simulink model "clc_sldv_m6"  (R2020b)
settings: Solver=ode3  StartTime=0.0  StopTime=simTime  FixedStep=0.01  RelTol=1e-6  AbsTol=1e-7
model workspace (MATLAB code in the model file):
  | % Load initial conditions and other information
  | 
  | load sldemo_clutchparam;
undefined symbols (not defined in the file): be, bv, DiscIntNeverNeededParam, Ie, Iv, muk, mus, R
Description:
  | Building a Clutch Lock-Up Model
  | 
  | This example demonstrates the use of Simulink to model and simulate a
  | rotating clutch system. Although modeling a clutch system is difficult
  | because of topological changes in the system dynamics during lockup, this
  | example shows how Simulinks enabled subsystems feature easily handles
  | such problems. We illustrate how to employ important Simulink modeling
  | concepts in the creation of the clutch simulation. Designers can apply
  | these concepts to many models with strong discontinuities and constraints
  | that may change dynamically.
  | 
  | In the demonstration, we use enabled subsystems to build the clutch
  | model. Two enabled subsystems model the clutch dynamics in either the
  | locked or unlocked position. After running the simulation, a GUI opens.
  | Checking any of the boxes on the GUI produces a plot of any of the
  | selected variables (versus time).
settings Model: ExtModeTrigMode=oneshot  ExtModeArmWhenConnect=off  ExtModeAutoUpdateStatusClock=off  Creator=The MathWorks Inc.  LastModifiedBy=Xiao Ling
settings SolverCC: AutoScaleAbsTol=off
settings DataIOCC: ExternalInput=externalinputdata  InitialState=[]  SaveFormat=Array  SignalLoggingSaveFormat=ModelDataLogs  SignalLogging=off  DSMLogging=off  ReturnWorkspaceOutputs=off  StateSaveName=x  SignalLoggingName=sldemo_clutch_output
settings OptimizationCC: BlockReduction=off  BooleanDataType=off  ExpressionDepthLimit=2147483647  InitFltsAndDblsToZero=on  LifeSpan=inf  BufferReusableBoundary=off
settings DebuggingCC: SaveWithParameterizedLinksMsg=none  UnderspecifiedInitializationDetection=Classic  MergeDetectMultiDrivingBlocksExec=none  SignalResolutionControl=TryResolveAllWithWarning  MultiTaskDSMMsg=warning  MultiTaskCondExecSysMsg=none  SigSpecEnsureSampleTimeMsg=none  IntegerOverflowMsg=none  FcnCallInpInsideContextMsg=warning  BusObjectLabelMismatch=none  StateNameClashWarn=warning  SFUnexpectedBacktrackingDiag=warning  SFNoUnconditionalDefaultTransitionDiag=warning  SFExecutionAtInitializationDiag=none  IntegerSaturationMsg=none  ArithmeticOperatorsInVariantConditions=warning
settings HardwareCC: ProdBitPerPointer=32  ProdBitPerSizeT=32  ProdBitPerPtrDiffT=32  ProdLargestAtomicFloat=None  ProdIntDivRoundTo=Undefined  ProdEndianess=Unspecified  ProdWordSize=32  ProdHWDeviceType=32-bit Generic  TargetUnknown=on
settings ModelReferenceCC: PropagateSignalLabelsOutOfModel=off
settings CodeAppCC: StateflowObjectComments=on
settings GRTTargetCC: TargetFcnLib=ansi_tfl_tmw.mat  TargetLangStandard=C89/C90 (ANSI)  CombineOutputUpdateFcns=off  GRTInterface=on
settings ConfigComp: CovMetricSettings=d  CovSaveCumulativeToWorkspaceVar=on  CovSaveSingleToWorkspaceVar=on  DVMaxProcessTime=600  DVParameters=on  DVModelCoverageObjectives=Decision  DVMaxTestCaseSteps=500  DVTestSuiteOptimization=CombinedObjectives  DVDetectActiveLogic=on  DVDetectOutOfBounds=on  DVSaveHarnessModel=on  DVSaveReport=on

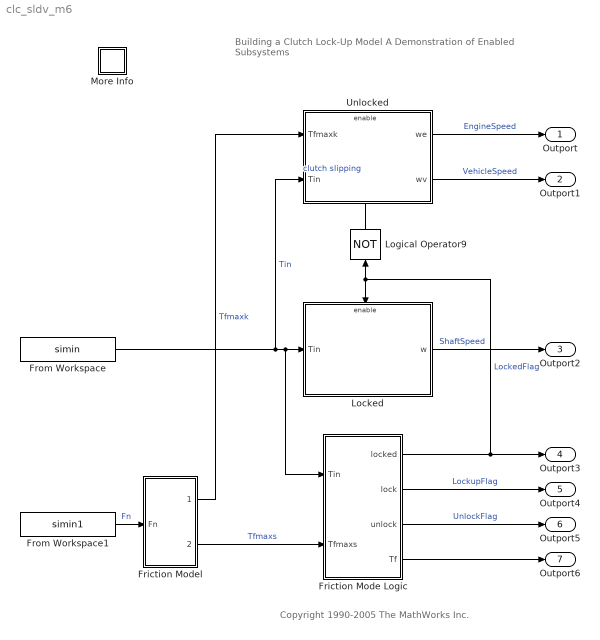
== system clc_sldv_m6 ==
  note: Building a Clutch Lock-Up Model
      | A Demonstration of Enabled Subsystems
  note: Copyright 1990-2005 The MathWorks Inc.
  Friction Model : Subsystem
  Friction Mode Logic : Subsystem
      mask Display: plot([-3 1 1 3 -1 -1],[-1 -1 1 1 1 -1],-4,-5,4,5)
  From Workspace : FromWorkspace  VariableName=simin
  From Workspace1 : FromWorkspace  VariableName=simin1
  Locked : Subsystem  TreatAsAtomicUnit=on
      mask Display: plot(-1,-6,6,12,[0 3],[3 3],[3 1 1 3], [1 1 5 5],[2 4 4 2],[4 4 2 2],[4 5],[3 3])
  Logical Operator9 : Logic  Operator=NOT  Inputs=1  IconShape=distinctive
  More Info : Subsystem
      settings: OpenFcn=showdemo(bdroot(gcb))
      mask Display: disp('?')
  Unlocked : Subsystem  TreatAsAtomicUnit=on
      mask Display: plot(-1,-2,6,8,[0 3],[3 3],[3 1 1 3], [1 1 5 5],[2 4 4 2],[4 4 2 2],[4 5],[3 3])
  Outport : Outport
  Outport1 : Outport  Port=2
  Outport2 : Outport  Port=3
  Outport3 : Outport  Port=4
  Outport4 : Outport  Port=5
  Outport5 : Outport  Port=6
  Outport6 : Outport  Port=7
  wires:
  Friction Mode Logic/3(unlock) -> Outport5/1  "UnlockFlag"
  From Workspace/1 -> Locked/1(Tin), Friction Mode Logic/1(Tin), Unlocked/2(Tin)  "Tin"
  Friction Model/1(Tfmaxk) -> Unlocked/1(Tfmaxk)  "Tfmaxk"
  Unlocked/2(wv) -> Outport1/1  "VehicleSpeed"
  Unlocked/1(we) -> Outport/1  "EngineSpeed"
  Friction Mode Logic/1(locked) -> Outport3/1, Logical Operator9/1, Locked/Enable  "LockedFlag"
  Friction Mode Logic/2(lock) -> Outport4/1  "LockupFlag"
  Friction Mode Logic/4(Tf) -> Outport6/1
  Locked/1(w) -> Outport2/1  "ShaftSpeed"
  Logical Operator9/1 -> Unlocked/Enable  "clutch slipping"
  Friction Model/2(Tfmaxs) -> Friction Mode Logic/2(Tfmaxs)  "Tfmaxs"
  From Workspace1/1 -> Friction Model/1(Fn)  "Fn"

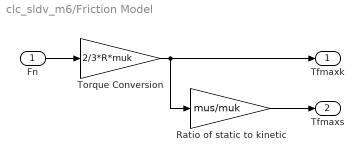
== system clc_sldv_m6/Friction Model ==
  Fn : Inport
  Ratio of static to kinetic : Gain  Gain=mus/muk  SaturateOnIntegerOverflow=on  OutDataTypeStr=Inherit: Same as input  ParamDataTypeStr=Inherit: Same as input
  Torque Conversion : Gain  Gain=2/3*R*muk  SaturateOnIntegerOverflow=on  OutDataTypeStr=Inherit: Same as input  ParamDataTypeStr=Inherit: Same as input
  Tfmaxk : Outport  InitialOutput=0
  Tfmaxs : Outport  Port=2  InitialOutput=0
  wires:
  Torque Conversion/1 -> Tfmaxk/1, Ratio of static to kinetic/1
  Fn/1 -> Torque Conversion/1
  Ratio of static to kinetic/1 -> Tfmaxs/1

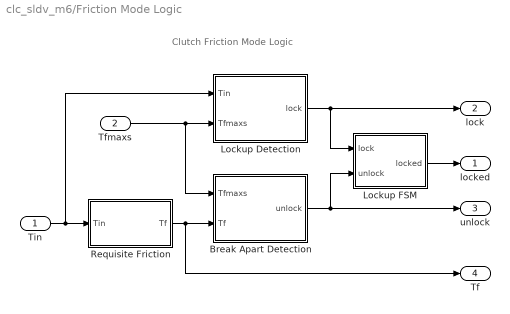
== system clc_sldv_m6/Friction Mode Logic ==
  note: Clutch Friction Mode Logic
  Tin : Inport
  Tfmaxs : Inport  Port=2
  Break Apart Detection : Subsystem
  Lockup Detection : Subsystem
  Lockup FSM : Subsystem
  Requisite Friction : Subsystem
  locked : Outport  InitialOutput=0
  lock : Outport  Port=2  InitialOutput=0
  unlock : Outport  Port=3  InitialOutput=0
  Tf : Outport  Port=4  InitialOutput=0
  wires:
  Tin/1 -> Lockup Detection/1(Tin), Requisite Friction/1(Tin)
  Tfmaxs/1 -> Lockup Detection/2(Tfmaxs), Break Apart Detection/1(Tfmaxs)
  Requisite Friction/1(Tf) -> Break Apart Detection/2(Tf), Tf/1
  Break Apart Detection/1(unlock) -> Lockup FSM/2(unlock), unlock/1
  Lockup Detection/1(lock) -> Lockup FSM/1(lock), lock/1
  Lockup FSM/1(locked) -> locked/1

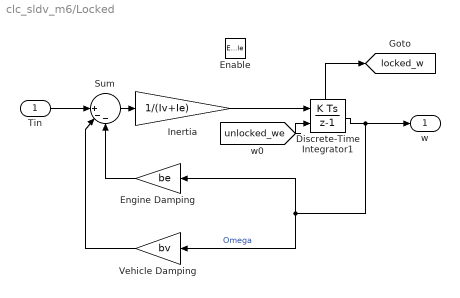
== system clc_sldv_m6/Locked ==
  Tin : Inport
  Enable : EnablePort  StatesWhenEnabling=reset
  Discrete-Time Integrator1 : DiscreteIntegrator  InitialConditionSource=external  ShowStatePort=on  ICPrevOutput=DiscIntNeverNeededParam  ICPrevScaledInput=DiscIntNeverNeededParam
  Engine Damping : Gain  Gain=be  SaturateOnIntegerOverflow=on  OutDataTypeStr=Inherit: Same as input  ParamDataTypeStr=Inherit: Same as input
  Inertia : Gain  Gain=1/(Iv+Ie)  SaturateOnIntegerOverflow=on  OutDataTypeStr=Inherit: Same as input  ParamDataTypeStr=Inherit: Same as input
  Sum : Sum  Inputs=||+--  InputSameDT=on  SaturateOnIntegerOverflow=on  OutDataTypeStr=Inherit: Same as first input
  Vehicle Damping : Gain  Gain=bv  SaturateOnIntegerOverflow=on  OutDataTypeStr=Inherit: Same as input  ParamDataTypeStr=Inherit: Same as input
  w : Outport  InitialOutput=0
  tag scope: locked_w=global
  wires:
  [unlocked_we] -> Discrete-Time Integrator1/2
  Discrete-Time Integrator1/State -> [locked_w]
  Sum/1 -> Inertia/1
  Tin/1 -> Sum/1
  Discrete-Time Integrator1/1 -> w/1, Engine Damping/1, Vehicle Damping/1  "Omega"
  Engine Damping/1 -> Sum/3
  Inertia/1 -> Discrete-Time Integrator1/1
  Vehicle Damping/1 -> Sum/2

== system clc_sldv_m6/More Info ==

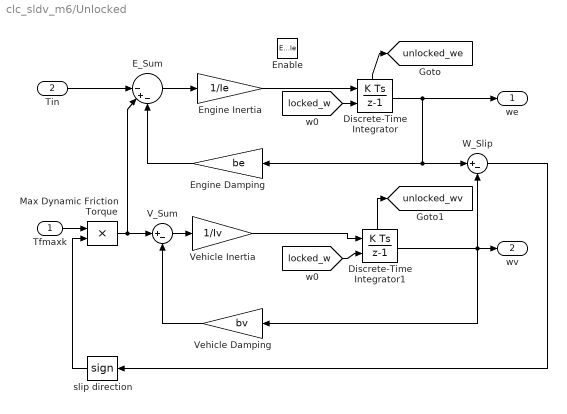
== system clc_sldv_m6/Unlocked ==
  Tfmaxk : Inport
  Tin : Inport  Port=2
  Enable : EnablePort  StatesWhenEnabling=reset
  Discrete-Time Integrator : DiscreteIntegrator  InitialConditionSource=external  ShowStatePort=on  ICPrevOutput=DiscIntNeverNeededParam  ICPrevScaledInput=DiscIntNeverNeededParam
  Discrete-Time Integrator1 : DiscreteIntegrator  InitialConditionSource=external  ShowStatePort=on  ICPrevOutput=DiscIntNeverNeededParam  ICPrevScaledInput=DiscIntNeverNeededParam
  E_Sum : Sum  Inputs=||-+-  InputSameDT=on  SaturateOnIntegerOverflow=on  OutDataTypeStr=Inherit: Same as first input
  Engine Damping : Gain  Gain=be  SaturateOnIntegerOverflow=on  OutDataTypeStr=Inherit: Same as input  ParamDataTypeStr=Inherit: Same as input
  Engine Inertia : Gain  Gain=1/Ie  SaturateOnIntegerOverflow=on  OutDataTypeStr=Inherit: Same as input  ParamDataTypeStr=Inherit: Same as input
  Max Dynamic Friction Torque : Product  InputSameDT=on  RndMeth=Zero  SaturateOnIntegerOverflow=on  OutDataTypeStr=Inherit: Same as first input
  V_Sum : Sum  Inputs=|+-  InputSameDT=on  SaturateOnIntegerOverflow=on  OutDataTypeStr=Inherit: Same as first input
  Vehicle Damping : Gain  Gain=bv  SaturateOnIntegerOverflow=on  OutDataTypeStr=Inherit: Same as input  ParamDataTypeStr=Inherit: Same as input
  Vehicle Inertia : Gain  Gain=1/Iv  SaturateOnIntegerOverflow=on  OutDataTypeStr=Inherit: Same as input  ParamDataTypeStr=Inherit: Same as input
  W_Slip : Sum  Inputs=|+-  InputSameDT=on  SaturateOnIntegerOverflow=on  OutDataTypeStr=Inherit: Same as first input
  slip direction : Signum
  we : Outport  InitialOutput=0
  wv : Outport  Port=2  InitialOutput=0
  tag scope: unlocked_we=global, unlocked_wv=global
  wires:
  V_Sum/1 -> Vehicle Inertia/1
  Vehicle Damping/1 -> V_Sum/2
  Max Dynamic Friction Torque/1 -> V_Sum/1, E_Sum/2
  Tfmaxk/1 -> Max Dynamic Friction Torque/1
  slip direction/1 -> Max Dynamic Friction Torque/2
  W_Slip/1 -> slip direction/1
  Discrete-Time Integrator/State -> [unlocked_we]
  Engine Inertia/1 -> Discrete-Time Integrator/1
  E_Sum/1 -> Engine Inertia/1
  Engine Damping/1 -> E_Sum/3
  Discrete-Time Integrator/1 -> we/1, Engine Damping/1, W_Slip/1
  [locked_w] -> Discrete-Time Integrator/2
  Tin/1 -> E_Sum/1
  Discrete-Time Integrator1/State -> [unlocked_wv]
  [locked_w] -> Discrete-Time Integrator1/2
  Vehicle Inertia/1 -> Discrete-Time Integrator1/1
  Discrete-Time Integrator1/1 -> wv/1, W_Slip/2, Vehicle Damping/1

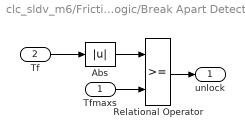
== system clc_sldv_m6/Friction Mode Logic/Break Apart Detection ==
  Tfmaxs : Inport
  Tf : Inport  Port=2
  Abs : Abs  SaturateOnIntegerOverflow=on
  Relational Operator : RelationalOperator  RndMeth=Nearest  InputSameDT=on
  unlock : Outport  InitialOutput=0
  wires:
  Tf/1 -> Abs/1
  Relational Operator/1 -> unlock/1
  Abs/1 -> Relational Operator/1
  Tfmaxs/1 -> Relational Operator/2

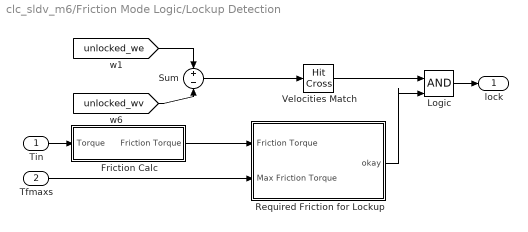
== system clc_sldv_m6/Friction Mode Logic/Lockup Detection ==
  Tin : Inport
  Tfmaxs : Inport  Port=2
  Friction Calc : Subsystem
  Logic : Logic  IconShape=distinctive
  Required Friction for Lockup : Subsystem
  Sum : Sum  Inputs=+-  InputSameDT=on  SaturateOnIntegerOverflow=on  OutDataTypeStr=Inherit: Same as first input
  Velocities Match : HitCross
  lock : Outport  InitialOutput=0
  wires:
  Friction Calc/1(Friction Torque) -> Required Friction for Lockup/1(Friction Torque)
  Tfmaxs/1 -> Required Friction for Lockup/2(Max Friction Torque)
  Velocities Match/1 -> Logic/1
  Logic/1 -> lock/1
  Required Friction for Lockup/1(okay) -> Logic/2
  [unlocked_we] -> Sum/1
  [unlocked_wv] -> Sum/2
  Sum/1 -> Velocities Match/1
  Tin/1 -> Friction Calc/1(Torque)

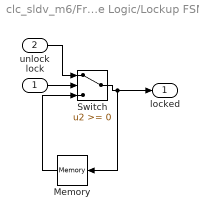
== system clc_sldv_m6/Friction Mode Logic/Lockup FSM ==
  lock : Inport
  unlock : Inport  Port=2
  Memory : Memory
  Switch : Switch
  locked : Outport  InitialOutput=0
  wires:
  Switch/1 -> locked/1, Memory/1
  lock/1 -> Switch/2
  Memory/1 -> Switch/3
  unlock/1 -> Switch/1

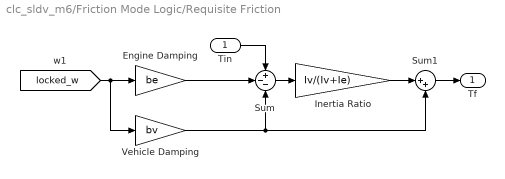
== system clc_sldv_m6/Friction Mode Logic/Requisite Friction ==
  Tin : Inport
  Engine Damping : Gain  Gain=be  SaturateOnIntegerOverflow=on  OutDataTypeStr=Inherit: Same as input  ParamDataTypeStr=Inherit: Same as input
  Inertia Ratio : Gain  Gain=Iv/(Iv+Ie)  SaturateOnIntegerOverflow=on  OutDataTypeStr=Inherit: Same as input  ParamDataTypeStr=Inherit: Same as input
  Sum : Sum  Inputs=+--  InputSameDT=on  SaturateOnIntegerOverflow=on  OutDataTypeStr=Inherit: Same as first input
  Sum1 : Sum  Inputs=|++  InputSameDT=on  SaturateOnIntegerOverflow=on  OutDataTypeStr=Inherit: Same as first input
  Vehicle Damping : Gain  Gain=bv  SaturateOnIntegerOverflow=on  OutDataTypeStr=Inherit: Same as input  ParamDataTypeStr=Inherit: Same as input
  Tf : Outport  InitialOutput=0
  wires:
  [locked_w] -> Vehicle Damping/1, Engine Damping/1
  Engine Damping/1 -> Sum/2
  Vehicle Damping/1 -> Sum/3, Sum1/2
  Sum/1 -> Inertia Ratio/1
  Tin/1 -> Sum/1
  Inertia Ratio/1 -> Sum1/1
  Sum1/1 -> Tf/1

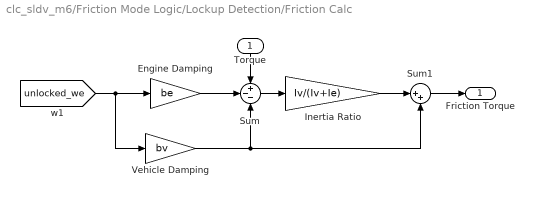
== system clc_sldv_m6/Friction Mode Logic/Lockup Detection/Friction Calc ==
  Torque : Inport
  Engine Damping : Gain  Gain=be  SaturateOnIntegerOverflow=on  OutDataTypeStr=Inherit: Same as input  ParamDataTypeStr=Inherit: Same as input
  Inertia Ratio : Gain  Gain=Iv/(Iv+Ie)  SaturateOnIntegerOverflow=on  OutDataTypeStr=Inherit: Same as input  ParamDataTypeStr=Inherit: Same as input
  Sum : Sum  Inputs=+--  InputSameDT=on  SaturateOnIntegerOverflow=on  OutDataTypeStr=Inherit: Same as first input
  Sum1 : Sum  Inputs=|++  InputSameDT=on  SaturateOnIntegerOverflow=on  OutDataTypeStr=Inherit: Same as first input
  Vehicle Damping : Gain  Gain=bv  SaturateOnIntegerOverflow=on  OutDataTypeStr=Inherit: Same as input  ParamDataTypeStr=Inherit: Same as input
  Friction Torque : Outport  InitialOutput=0
  wires:
  [unlocked_we] -> Engine Damping/1, Vehicle Damping/1
  Vehicle Damping/1 -> Sum1/2, Sum/3
  Engine Damping/1 -> Sum/2
  Sum/1 -> Inertia Ratio/1
  Torque/1 -> Sum/1
  Inertia Ratio/1 -> Sum1/1
  Sum1/1 -> Friction Torque/1

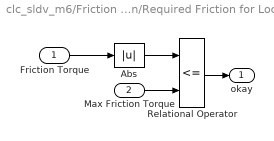
== system clc_sldv_m6/Friction Mode Logic/Lockup Detection/Required Friction for Lockup ==
  Friction Torque : Inport
  Max Friction Torque : Inport  Port=2
  Abs : Abs  SaturateOnIntegerOverflow=on
  Relational Operator : RelationalOperator  Operator=<=  RndMeth=Nearest  InputSameDT=on
  okay : Outport  InitialOutput=0
  wires:
  Friction Torque/1 -> Abs/1
  Relational Operator/1 -> okay/1
  Abs/1 -> Relational Operator/1
  Max Friction Torque/1 -> Relational Operator/2
